simulink model "Esempiobatteria"  (R2023b)
settings: Solver=VariableStepAuto  StartTime=0.0  StopTime=10.0  RelTol=1e-3
undefined symbols (not defined in the file): R0, soc0
libraries: autolibdatasheetbattery x1, autolibrcnetworksystem x1
settings Model: Creator=elis  LastModifiedBy=chris
settings OptimizationCC: ReuseModelBlockBuffer=off

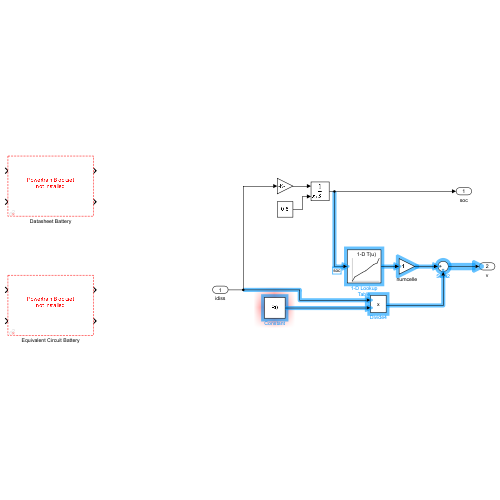
[thumbnail: Simulink's stored preview of the top-level diagram]
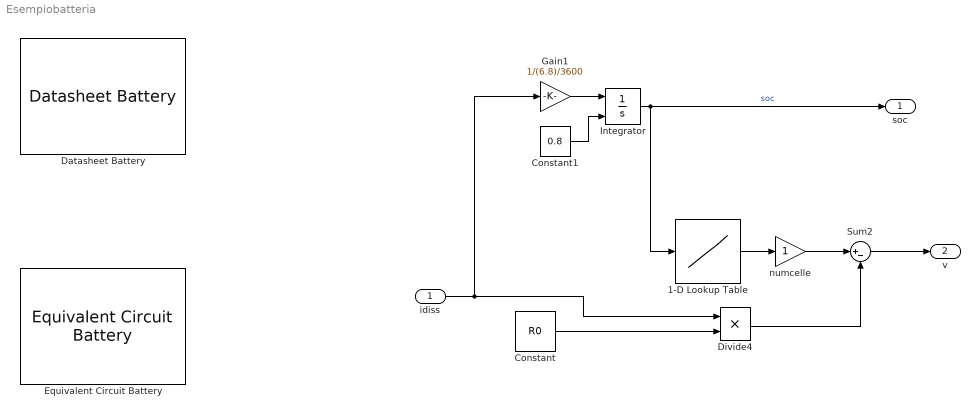
== system Esempiobatteria ==
  idiss : Inport
  1-D Lookup Table : Lookup_n-D  NumberOfTableDimensions=1  BreakpointsForDimension1=[0, .1, .38,.511,.8,.92, 1]  Table=[3.28, 3.45, 3.63, 3.69,3.95,4.01,4.2]  InternalRulePriority=Speed  RndMeth=Simplest
  Constant : Constant  Value=R0
  Constant1 : Constant  Value=0.8
  Datasheet Battery : autolibdatasheetbattery/Datasheet Battery  CapacityCtrl=Parameter  OutputVlt=Unfiltered  BattChargeMax=100  Em=[2.8 3.228 3.284 3.361 3.408 3.427 3.472 3.477 3.493 3.504 3.516 3.528 3.537 3.545 3.555 3.561 3.566 3.576 3.587 3.589 3.594 3.6 3.608 3.61 3.616 3.619 3.626 3.632 3.637 3.64 3.645 3.646 3.652 3.655 3.658 3.661 3.664 3.668 3.673 3.678 3.68 3.681 3.686 3.692 3.699 3.702 3.705 3.71 3.717 3.723 3.728 3.733 3.735 3.742 3.749 3.755 3.761 3.768 3.773 3.78 3.791 3.798 3.798 3.814 3.818 3.825 3.841 3.846 3.855 3.863 3.877 3.885 3.894 3.907 3.919 3.926 3.935 3.944 3.954 3.964 3.974 3.988 3.998 4.014 4.029 4.034 4.047 4.065 4.074 4.086 4.097 4.131 4.126 4.138 4.15 4.18 4.174 4.187 4.207 4.231 4.221]  CapLUTBp=[0 0.01 0.02 0.03 0.04 0.05 0.06 0.07 0.08 0.09 0.1 0.11 0.12 0.13 0.14 0.15 0.16 0.17 0.18 0.19 0.2 0.21 0.22 0.23 0.24 0.25 0.26 0.27 0.28 0.29 0.3 0.31 0.32 0.33 0.34 0.35 0.36 0.37 0.38 0.39 0.4 0.41 0.42 0.43 0.44 0.45 0.46 0.47 0.48 0.49 0.5 0.51 0.52 0.53 0.54 0.55 0.56 0.57 0.58 0.59 0.6 0.61 0.62 0.63 0.64 0.65 0.66 0.67 0.68 0.69 0.7 0.71 0.72 0.73 0.74 0.75 0.76 0.77 0.78 0.79 0.8 0.81 0.82 0.83 0.84 0.85 0.86 0.87 0.88 0.89 0.9 0.91 0.92 0.93 0.94 0.95 0.96 0.97 0.98 0.99 1]  RInt=[0.008846 0.009319 0.009027 0.00847 0.01032 0.01314;0.006389 0.006554 0.005553 0.005525 0.006043 0.007805;0.004364 0.004101 0.00406 0.003452 0.003846 0.004517;0.002031 0.002563 0.002532 0.00246 0.002716 0.003047;0.001443 0.001825 0.001795 0.001778 0.001924 0.002234;0.0005603 0.0007192 0.0006887 0.0007557 0.0007355 0.001014;0.001028 0.001338 0.001 0.001536 0.001546 0.002789]  BattTempBp=[243.1 253.1 263.1 273.1 283.1 298.1 313.1]  CapSOCBp=[0 0.2 0.4 0.6 0.8 1]  Ns=1  Np=1  BattCapInit=100  Tc=1/1000  Vinit=4.221  RefBlkName='autolibdatasheetbattery/Datasheet Battery'
  Divide4 : Product  Inputs=**
  Equivalent Circuit Battery : autolibrcnetworksystem/Equivalent Circuit Battery  CapacityCtrl=Parameter  OutputVlt=Unfiltered  NumRC=1  Em=|  R0=|  SOC_BP=|  Temperature_BP=[293.15 313.15]  BattCap=[28 28]  BattCapInit=28  InitialCapVoltage=0  Tc=1/1000  Vinit=4.193  R1=|  C1=|  R2=|  C2=|  R3=|  C3=|  R4=|  C4=|  R5=|  C5=|  Vu=Inf  Vl=-Inf  RefBlkName='autolibrcnetworksystem/Equivalent Circuit Battery'
      Em=|
      | [3.5042 3.5136;
      | 3.5573 3.5646;
      | 3.6009 3.6153;
      | 3.6393 3.6565;
      | 3.6742 3.6889;
      | 3.7121 3.7214;
      | 3.7937 3.8078;
      | 3.8753 3.8945;
      | 3.97 3.9859;
      | 4.0764 4.0821;
      | 4.1924 4.193]
      R0=|
      | [0.011448 0.0090006;
      | 0.011038 0.0089655;
      | 0.011281 0.0091261;
      | 0.011236 0.0091099;
      | 0.010959 0.008957;
      | 0.010714 0.0087969;
      | 0.010698 0.0089126;
      | 0.010712 0.0090517;
      | 0.010917 0.0090444;
      | 0.011304 0.0088992;
      | 0.011603 0.0089015
      | ]
      SOC_BP=|
      | [0
      | 0.1
      | 0.2
      | 0.3
      | 0.4
      | 0.5
      | 0.6
      | 0.7
      | 0.8
      | 0.9
      | 1]
      R1=|
      | [0.010342 0.0012244;
      | 0.0067316 0.0011396;
      | 0.0051156 0.0012661;
      | 0.0043447 0.0012265;
      | 0.0038826 0.0011163;
      | 0.0034226 0.0009968;
      | 0.003346 0.0011458;
      | 0.0033222 0.001345;
      | 0.0033201 0.0013091;
      | 0.0032886 0.0010986;
      | 0.0028114 0.0010309]
      C1=|
      | [2287.7 11897;
      | 6122 24515;
      | 18460 42098;
      | 20975 44453;
      | 15254 33098;
      | 10440 24492;
      | 13903 32975;
      | 16694 40007;
      | 15784 35937;
      | 12165 26430;
      | 9118 24795]
      R2=|
      | [0.010342 0.0012244;
      | 0.0067316 0.0011396;
      | 0.0051156 0.0012661;
      | 0.0043447 0.0012265;
      | 0.0038826 0.0011163;
      | 0.0034226 0.0009968;
      | 0.003346 0.0011458;
      | 0.0033222 0.001345;
      | 0.0033201 0.0013091;
      | 0.0032886 0.0010986;
      | 0.0028114 0.0010309]
      C2=|
      | [2287.7 11897;
      | 6122 24515;
      | 18460 42098;
      | 20975 44453;
      | 15254 33098;
      | 10440 24492;
      | 13903 32975;
      | 16694 40007;
      | 15784 35937;
      | 12165 26430;
      | 9118 24795]
      R3=|
      | [0.010342 0.0012244;
      | 0.0067316 0.0011396;
      | 0.0051156 0.0012661;
      | 0.0043447 0.0012265;
      | 0.0038826 0.0011163;
      | 0.0034226 0.0009968;
      | 0.003346 0.0011458;
      | 0.0033222 0.001345;
      | 0.0033201 0.0013091;
      | 0.0032886 0.0010986;
      | 0.0028114 0.0010309]
      C3=|
      | [2287.7 11897;
      | 6122 24515;
      | 18460 42098;
      | 20975 44453;
      | 15254 33098;
      | 10440 24492;
      | 13903 32975;
      | 16694 40007;
      | 15784 35937;
      | 12165 26430;
      | 9118 24795]
      R4=|
      | [0.010342 0.0012244;
      | 0.0067316 0.0011396;
      | 0.0051156 0.0012661;
      | 0.0043447 0.0012265;
      | 0.0038826 0.0011163;
      | 0.0034226 0.0009968;
      | 0.003346 0.0011458;
      | 0.0033222 0.001345;
      | 0.0033201 0.0013091;
      | 0.0032886 0.0010986;
      | 0.0028114 0.0010309]
      C4=|
      | [2287.7 11897;
      | 6122 24515;
      | 18460 42098;
      | 20975 44453;
      | 15254 33098;
      | 10440 24492;
      | 13903 32975;
      | 16694 40007;
      | 15784 35937;
      | 12165 26430;
      | 9118 24795]
      R5=|
      | [0.010342 0.0012244;
      | 0.0067316 0.0011396;
      | 0.0051156 0.0012661;
      | 0.0043447 0.0012265;
      | 0.0038826 0.0011163;
      | 0.0034226 0.0009968;
      | 0.003346 0.0011458;
      | 0.0033222 0.001345;
      | 0.0033201 0.0013091;
      | 0.0032886 0.0010986;
      | 0.0028114 0.0010309]
      C5=|
      | [2287.7 11897;
      | 6122 24515;
      | 18460 42098;
      | 20975 44453;
      | 15254 33098;
      | 10440 24492;
      | 13903 32975;
      | 16694 40007;
      | 15784 35937;
      | 12165 26430;
      | 9118 24795]
  Gain1 : Gain  Gain=1/(6.8)/3600
  Integrator : Integrator  InitialConditionSource=external  InitialCondition=soc0
  Sum2 : Sum  Inputs=|+-
  numcelle : Gain
  soc : Outport
  v : Outport  Port=2
  wires:
  Gain1/1 -> Integrator/1
  Integrator/1 -> 1-D Lookup Table/1, soc/1  "soc"
  Sum2/1 -> v/1
  Divide4/1 -> Sum2/2
  numcelle/1 -> Sum2/1
  Constant1/1 -> Integrator/2
  Constant/1 -> Divide4/2
  1-D Lookup Table/1 -> numcelle/1
  idiss/1 -> Gain1/1, Divide4/1
